simulink subsystem "EV3_Logic"  (R2020a)
settings: Solver=VariableStepAuto  StartTime=0.0  StopTime=10.0  RelTol=1e-3
values from neighbouring files (symbols this model uses):
  track = [1.6187 1.6087 1.5987 1.5887 1.5787 1.5687 1.5587 1.5487 1.5387 1.5287 1.5187 1.5087 ... (4048 elements, 1012x4)]    [config.mat]    (also in gen_track.m = [line_b; turn_bl; line_l; turn_lc; line_c; turn_ct; line_t; )
libraries: simulink_extras x5, simulink x4, dspnetwork x4, fuzblock x2
settings Model: Creator=Duncan  LastModifiedBy=abatra2

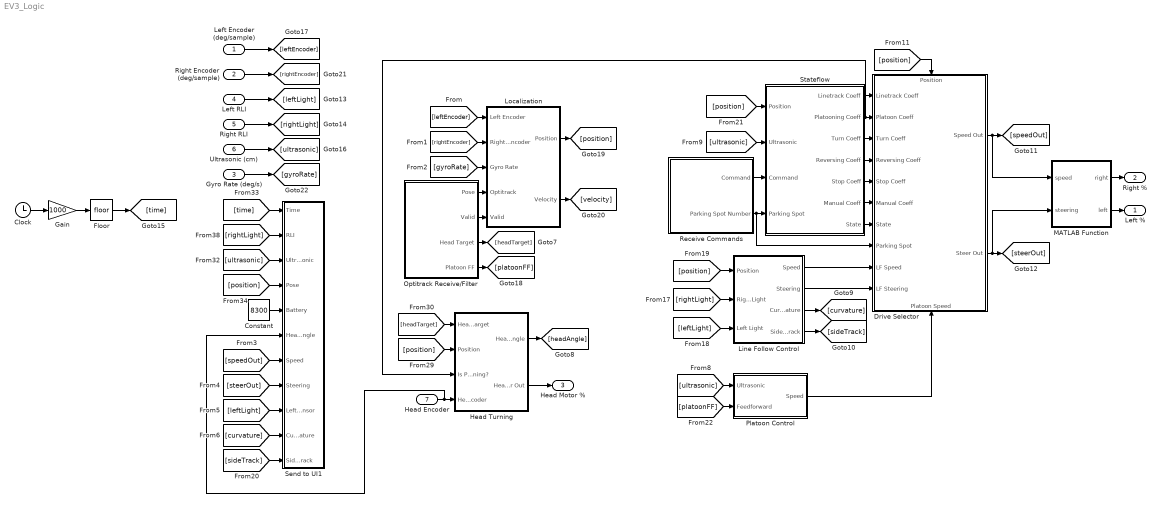
== system EV3_Logic ==
  Left Encoder (deg/sample) : Inport
  Right Encoder (deg/sample) : Inport  Port=2
  Gyro Rate (deg/s) : Inport  Port=3
  Left RLI : Inport  Port=4
  Right RLI : Inport  Port=5
  Ultrasonic (cm) : Inport  Port=6
  Head Encoder : Inport  Port=7
  Clock : Clock
  Constant : Constant  Value=8300
  Drive Selector : Subsystem
      settings: PortSchema="{\"entries\":[{\"content\":{\"sides\":[{\"content\":{\"connectorIds\":[\"In1\",\"In2\",\"In3\",\"In4\",\"In5\",\"In6\",\"In7\",\"In8\",\"In9\",\"In10\"]},\"type\":\"ConnectorPlacement.EquallySpacedRectSide\",\"uuid\":\"ae307232-287c-4602-bc59-e7aee20cf720\"},{\"content\":{\"connectorIds\":[\"Out1\",\"Out2\"],\"side\":\"RIGHT\"},\"type\":\"ConnectorPlacement.EquallySpacedRectSide\",\"uuid\":\"2cae2544-d808-4029-9530-a1f56251b9cd\"},{\"content\":{\"connectorIds\":[\"In11\"],\"side\":\"TOP\"},\"type\":\"ConnectorPlacement.EquallySpacedRectSide\",\"uuid\":\"bbc0be7b-0147-487e-824e-99eef1e06dcc\"},{\"content\":{\"connectorIds\":[\"In12\"],\"side\":\"BOTTOM\"},\"type\":\"ConnectorPlacement.EquallySpacedRectSide\",\"uuid\":\"b1fbed80-afe2-48db-af11-c85938407aae\"}]},\"type\":\"ConnectorPlacement.EquallySpacedConnector\",\"uuid\":\"38f7d747-6147-4f1b-8575-02c2e0fe0660\"}],\"packageUris\":[\"http://schema.mathworks.com/mf0/Connector/19700101\"],\"version\":\"1.0\"}"
  Floor : Rounding
  Gain : Gain  Gain=1000
  Head Turning : Subsystem
  Line Follow Control : Subsystem
  Localization : Subsystem
  MATLAB Function : MATLAB Function  TreatAsAtomicUnit=on
  Optitrack Receive/Filter : Subsystem
  Platoon Control : Subsystem
  Receive Commands : Subsystem
  Send to UI1 : Subsystem
  Stateflow : Subsystem
  Left % : Outport
  Right % : Outport  Port=2
  Head Motor % : Outport  Port=3
  wires:
  Ultrasonic (cm)/1 -> [ultrasonic]
  Right RLI/1 -> [rightLight]
  Left Encoder (deg/sample)/1 -> [leftEncoder]
  Right Encoder (deg/sample)/1 -> [rightEncoder]
  Left RLI/1 -> [leftLight]
  Gyro Rate (deg/s)/1 -> [gyroRate]
  Drive Selector/1(Speed Out) -> MATLAB Function/1(speed), [speedOut]
  Drive Selector/2(Steer Out) -> MATLAB Function/2(steering), [steerOut]
  Platoon Control/1(Speed) -> Drive Selector/12(Platoon Speed)
  Line Follow Control/4(Side Track) -> [sideTrack]
  Line Follow Control/3(Curvature) -> [curvature]
  Line Follow Control/2(Steering) -> Drive Selector/10(LF Steering)
  Line Follow Control/1(Speed) -> Drive Selector/9(LF Speed)
  Stateflow/2(Platooning Coeff) -> Drive Selector/2(Platoon Coeff), Head Turning/3(Is Platooning?)
  [ultrasonic] -> Platoon Control/1(Ultrasonic)
  [platoonFF] -> Platoon Control/2(Feedforward)
  Receive Commands/2(Parking Spot Number) -> Stateflow/4(Parking Spot), Drive Selector/8(Parking Spot)
  [ultrasonic] -> Stateflow/2(Ultrasonic)
  [position] -> Stateflow/1(Position)
  [sideTrack] -> Send to UI1/11(Side Track)
  [curvature] -> Send to UI1/10(Curvature)
  [leftLight] -> Send to UI1/9(Left Sensor)
  [steerOut] -> Send to UI1/8(Steering)
  [speedOut] -> Send to UI1/7(Speed)
  [position] -> Send to UI1/4(Pose)
  Stateflow/3(Turn Coeff) -> Drive Selector/3(Turn Coeff)
  [position] -> Drive Selector/11(Position)
  Localization/1(Position) -> [position]
  [leftEncoder] -> Localization/1(Left Encoder)
  Head Turning/1(Head Angle) -> [headAngle]
  Optitrack Receive/Filter/1(Pose) -> Localization/4(Optitrack)
  Stateflow/7(State) -> Drive Selector/7(State)
  Stateflow/5(Stop Coeff) -> Drive Selector/5(Stop Coeff)
  [rightEncoder] -> Localization/2(Right Encoder)
  [leftLight] -> Line Follow Control/3(Left Light)
  Stateflow/4(Reversing Coeff) -> Drive Selector/4(Reversing Coeff)
  [position] -> Head Turning/2(Position)
  [rightLight] -> Send to UI1/2(RLI)
  Localization/2(Velocity) -> [velocity]
  [time] -> Send to UI1/1(Time)
  [headTarget] -> Head Turning/1(Head Target)
  [ultrasonic] -> Send to UI1/3(Ultrasonic)
  Stateflow/1(Linetrack Coeff) -> Drive Selector/1(Linetrack Coeff)
  Optitrack Receive/Filter/2(Valid) -> Localization/5(Valid)
  [rightLight] -> Line Follow Control/2(Right Light)
  [gyroRate] -> Localization/3(Gyro Rate)
  Receive Commands/1(Command) -> Stateflow/3(Command)
  Head Turning/2(Head Motor Out) -> Head Motor %/1
  Head Encoder/1 -> Head Turning/4(Head Encoder), Send to UI1/6(Head Angle)
  Clock/1 -> Gain/1
  Gain/1 -> Floor/1
  Floor/1 -> [time]
  Optitrack Receive/Filter/3(Head Target) -> [headTarget]
  [position] -> Line Follow Control/1(Position)
  Optitrack Receive/Filter/4(Platoon FF) -> [platoonFF]
  Stateflow/6(Manual Coeff) -> Drive Selector/6(Manual Coeff)
  MATLAB Function/1(right) -> Right %/1
  MATLAB Function/2(left) -> Left %/1
  Constant/1 -> Send to UI1/5(Battery)

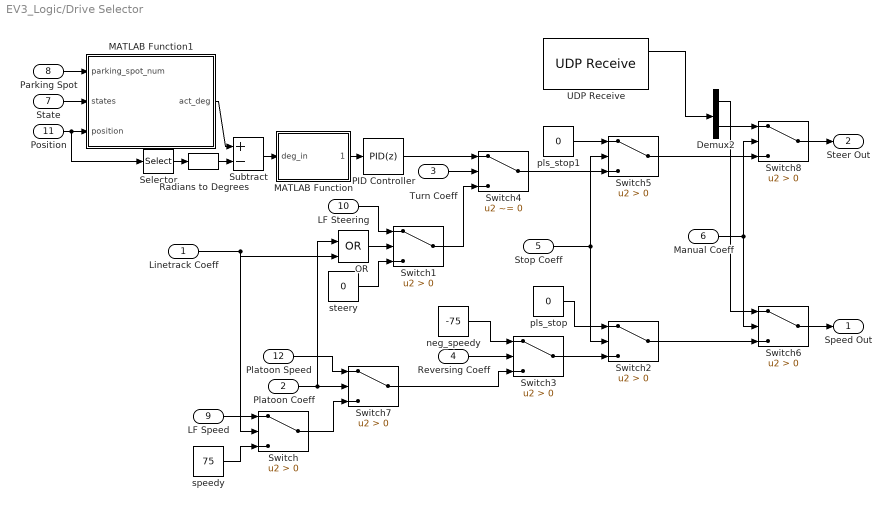
== system EV3_Logic/Drive Selector ==
  Linetrack Coeff : Inport
  Platoon Coeff : Inport  Port=2
  Turn Coeff : Inport  Port=3
  Reversing Coeff : Inport  Port=4
  Stop Coeff : Inport  Port=5
  Manual Coeff : Inport  Port=6
  State : Inport  Port=7
  Parking Spot : Inport  Port=8
  LF Speed : Inport  Port=9
  LF Steering : Inport  Port=10
  Position : Inport  Port=11
  Platoon Speed : Inport  Port=12
  Demux2 : Demux  Outputs=2
  MATLAB Function : MATLAB Function  TreatAsAtomicUnit=on
  MATLAB Function1 : MATLAB Function  TreatAsAtomicUnit=on
  OR : Logic  Operator=OR  IconShape=distinctive  AllPortsSameDT=off  OutDataTypeStr=boolean
  PID Controller : simulink/Continuous/PID Controller  Controller=PID  Form=Parallel  TimeDomain=Discrete-time  UseExternalTs=off  SampleTime=-1  IntegratorMethod=Forward Euler  FilterMethod=Forward Euler  ControllerParametersSource=internal  P=1  I=0  D=0  UseFilter=off  N=100  TunerSelectOption=Transfer Function Based (PID Tuner App)  InitialConditionSource=internal  InitialConditionForIntegrator=0  InitialConditionForFilter=0  DifferentiatorICPrevScaledInput=0  ExternalReset=none  TrackingMode=off  Kt=1  LimitOutput=off  UpperSaturationLimit=inf  LowerSaturationLimit=-inf  LinearizeAsGain=on  AntiWindupMode=none  Kb=1  POutMin=[]  POutMax=[]  IOutMin=[]  IOutMax=[]  DOutMin=[]  DOutMax=[]  NOutMin=[]  NOutMax=[]  SumOutMin=[]  SumOutMax=[]  SaturationOutMin=[]  SaturationOutMax=[]  PParamMin=[]  PParamMax=[]  IParamMin=[]  IParamMax=[]  DParamMin=[]  DParamMax=[]  NParamMin=[]  NParamMax=[]  KbParamMin=[]  KbParamMax=[]  KtParamMin=[]  KtParamMax=[]  KbOutMin=[]  KbOutMax=[]  KtOutMin=[]  KtOutMax=[]  IntegratorOutMin=[]  IntegratorOutMax=[]  FilterOutMin=[]  FilterOutMax=[]  SumI1OutMin=[]  SumI1OutMax=[]  SumI2OutMin=[]  SumI2OutMax=[]  SumI3OutMin=[]  SumI3OutMax=[]  SumI4OutMin=[]  SumI4OutMax=[]  SumDOutMin=[]  SumDOutMax=[]  DifferentiatorOutMin=[]  DifferentiatorOutMax=[]  FilterDiffOutCoefMin=[]  FilterDiffOutCoefMax=[]  ReciprocalOutMin=[]  ReciprocalOutMax=[]  SumDenOutMin=[]  SumDenOutMax=[]  SumNumOutMin=[]  SumNumOutMax=[]  DivideOutMin=[]  DivideOutMax=[]  UdiffTsProdOutMin=[]  UdiffTsProdOutMax=[]  NTsProdOutMin=[]  NTsProdOutMax=[]  UintegralTsProdOutMin=[]  UintegralTsProdOutMax=[]  UngainTsProdOutMin=[]  UngainTsProdOutMax=[]  IntegratorContinuousStateAttributes=''  IntegratorStateMustResolveToSignalObject=off  IntegratorRTWStateStorageClass=Auto  FilterContinuousStateAttributes=''  FilterStateMustResolveToSignalObject=off  FilterRTWStateStorageClass=Auto  ParallelPVariant=InternalParameters  IdealPVariant=Disabled  IVariant=InternalParameters  DVariant=InternalParameters  IntegratorVariant=Discrete  SatVariant=Disabled  AWVariant=Passthrough  PCopyVariant=Disabled  TRVariant=Disabled  FdbkBlocksVariant=Forward  IdealPFdbkVariant=Disabled  SatFdbkVariant=Disabled  DerivativeFilterVariant=Differentiator  NVariant=Passthrough  NCopyVariant=Disabled_SignalSpec  FilterICVariant=InternalICsDifferentiator  IntegratorICVariant=InternalICs  ExternalResetVariant=Disabled  TRSumVariant=Passthrough  SumFdbkVariant=Disabled  SumVariant=Sum_PID  TsampFilterVariant=InternalTs  TsampNgainVariant=Passthrough  TsampIntegralVariant=Passthrough
  Radians to Degrees : simulink_extras/Transformations/Radians to Degrees
  Selector : Selector  InputPortWidth=3  IndexOptions=Index vector (dialog)  Indices=[3]  OutputSizes=1
  Subtract : Sum  Inputs=+-
  Switch{,1..3,5..8} (8 alike) : Switch  Criteria=u2 > Threshold
  Switch4 : Switch  Criteria=u2 ~= 0
  UDP Receive : dspnetwork/UDP Receive  localURL='0.0.0.0'  localPort=joystickRXPort  remoteURL='0.0.0.0'  remotePort=-1  recvBufferSize=384  dims=2  signalDatatype=single  isComplex=off  isVarSize=off  showBlockingTime=off  blockingTime=0  sampletime=0.01  blockPlatform=[]
  neg_speedy : Constant  Value=-75
  pls_stop : Constant  Value=0
  pls_stop1 : Constant  Value=0
  speedy : Constant  Value=75
  steery : Constant  Value=0
  Speed Out : Outport
  Steer Out : Outport  Port=2
  wires:
  Platoon Speed/1 -> Switch7/1
  pls_stop1/1 -> Switch5/1
  Selector/1 -> Radians to Degrees/1
  Switch/1 -> Switch7/3
  Switch7/1 -> Switch3/3
  Linetrack Coeff/1 -> OR/2, Switch/2
  Platoon Coeff/1 -> Switch7/2, OR/1
  OR/1 -> Switch1/2
  MATLAB Function1/1(act_deg) -> Subtract/1
  neg_speedy/1 -> Switch3/1
  Switch4/1 -> Switch5/3
  Position/1 -> MATLAB Function1/3(position), Selector/1
  State/1 -> MATLAB Function1/2(states)
  Reversing Coeff/1 -> Switch3/2
  Parking Spot/1 -> MATLAB Function1/1(parking_spot_num)
  Radians to Degrees/1 -> Subtract/2
  MATLAB Function/1(deg_out) -> PID Controller/1
  Subtract/1 -> MATLAB Function/1(deg_in)
  PID Controller/1 -> Switch4/1
  Turn Coeff/1 -> Switch4/2
  pls_stop/1 -> Switch2/1
  Stop Coeff/1 -> Switch5/2, Switch2/2
  Switch3/1 -> Switch2/3
  Switch1/1 -> Switch4/3
  speedy/1 -> Switch/3
  steery/1 -> Switch1/3
  LF Steering/1 -> Switch1/1
  LF Speed/1 -> Switch/1
  UDP Receive/1 -> Demux2/1
  Switch5/1 -> Switch8/3
  Switch2/1 -> Switch6/3
  Manual Coeff/1 -> Switch8/2, Switch6/2
  Switch8/1 -> Steer Out/1
  Switch6/1 -> Speed Out/1
  Demux2/2 -> Switch8/1
  Demux2/1 -> Switch6/1

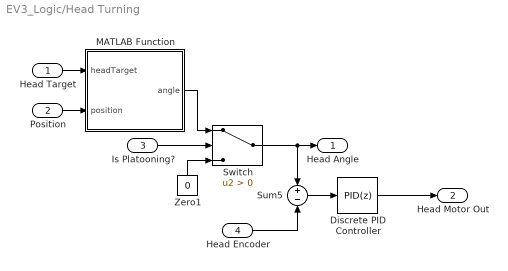
== system EV3_Logic/Head Turning ==
  Head Target : Inport
  Position : Inport  Port=2
  Is Platooning? : Inport  Port=3
  Head Encoder : Inport  Port=4
  Discrete PID Controller : simulink/Continuous/PID Controller  Controller=PID  Form=Parallel  TimeDomain=Discrete-time  UseExternalTs=off  SampleTime=-1  IntegratorMethod=Forward Euler  FilterMethod=Forward Euler  ControllerParametersSource=internal  P=1  I=1  D=0  UseFilter=off  N=100  TunerSelectOption=Transfer Function Based (PID Tuner App)  InitialConditionSource=internal  InitialConditionForIntegrator=0  InitialConditionForFilter=0  DifferentiatorICPrevScaledInput=0  ExternalReset=none  TrackingMode=off  Kt=1  LimitOutput=off  UpperSaturationLimit=inf  LowerSaturationLimit=-inf  LinearizeAsGain=off  AntiWindupMode=none  Kb=1  POutMin=[]  POutMax=[]  IOutMin=[]  IOutMax=[]  DOutMin=[]  DOutMax=[]  NOutMin=[]  NOutMax=[]  SumOutMin=[]  SumOutMax=[]  SaturationOutMin=[]  SaturationOutMax=[]  PParamMin=[]  PParamMax=[]  IParamMin=[]  IParamMax=[]  DParamMin=[]  DParamMax=[]  NParamMin=[]  NParamMax=[]  KbParamMin=[]  KbParamMax=[]  KtParamMin=[]  KtParamMax=[]  KbOutMin=[]  KbOutMax=[]  KtOutMin=[]  KtOutMax=[]  IntegratorOutMin=[]  IntegratorOutMax=[]  FilterOutMin=[]  FilterOutMax=[]  SumI1OutMin=[]  SumI1OutMax=[]  SumI2OutMin=[]  SumI2OutMax=[]  SumI3OutMin=[]  SumI3OutMax=[]  SumI4OutMin=[]  SumI4OutMax=[]  SumDOutMin=[]  SumDOutMax=[]  DifferentiatorOutMin=[]  DifferentiatorOutMax=[]  FilterDiffOutCoefMin=[]  FilterDiffOutCoefMax=[]  ReciprocalOutMin=[]  ReciprocalOutMax=[]  SumDenOutMin=[]  SumDenOutMax=[]  SumNumOutMin=[]  SumNumOutMax=[]  DivideOutMin=[]  DivideOutMax=[]  UdiffTsProdOutMin=[]  UdiffTsProdOutMax=[]  NTsProdOutMin=[]  NTsProdOutMax=[]  UintegralTsProdOutMin=[]  UintegralTsProdOutMax=[]  UngainTsProdOutMin=[]  UngainTsProdOutMax=[]  IntegratorContinuousStateAttributes=''  IntegratorStateMustResolveToSignalObject=off  IntegratorRTWStateStorageClass=Auto  FilterContinuousStateAttributes=''  FilterStateMustResolveToSignalObject=off  FilterRTWStateStorageClass=Auto  ParallelPVariant=InternalParameters  IdealPVariant=Disabled  IVariant=InternalParameters  DVariant=InternalParameters  IntegratorVariant=Discrete  SatVariant=Disabled  AWVariant=Passthrough  PCopyVariant=Disabled  TRVariant=Disabled  FdbkBlocksVariant=Forward  IdealPFdbkVariant=Disabled  SatFdbkVariant=Disabled  DerivativeFilterVariant=Differentiator  NVariant=Passthrough  NCopyVariant=Disabled_SignalSpec  FilterICVariant=InternalICsDifferentiator  IntegratorICVariant=InternalICs  ExternalResetVariant=Disabled  TRSumVariant=Passthrough  SumFdbkVariant=Disabled  SumVariant=Sum_PID  TsampFilterVariant=InternalTs  TsampNgainVariant=Passthrough  TsampIntegralVariant=Passthrough
  MATLAB Function : MATLAB Function  TreatAsAtomicUnit=on
  Sum5 : Sum  Inputs=+|-
  Switch : Switch  Criteria=u2 > Threshold
  Zero1 : Constant  Value=0  OutDataTypeStr=Inherit: Inherit via back propagation
  Head Angle : Outport
  Head Motor Out : Outport  Port=2
  wires:
  Is Platooning?/1 -> Switch/2
  MATLAB Function/1(angle) -> Switch/1
  Head Target/1 -> MATLAB Function/1(headTarget)
  Discrete PID Controller/1 -> Head Motor Out/1
  Switch/1 -> Sum5/1, Head Angle/1
  Zero1/1 -> Switch/3
  Sum5/1 -> Discrete PID Controller/1
  Position/1 -> MATLAB Function/2(position)
  Head Encoder/1 -> Sum5/2

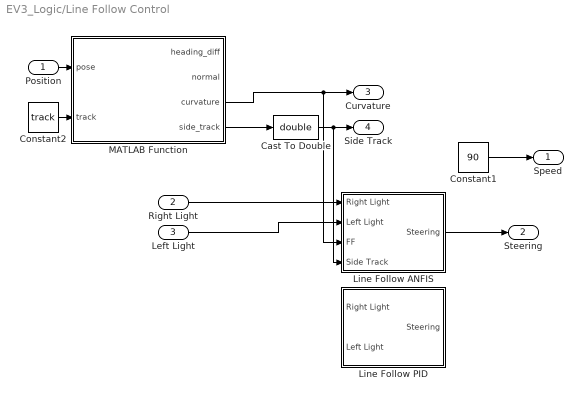
== system EV3_Logic/Line Follow Control ==
  Position : Inport
  Right Light : Inport  Port=2
  Left Light : Inport  Port=3
  Cast To Double : DataTypeConversion  OutDataTypeStr=double
  Constant1 : Constant  Value=90
  Constant2 : Constant  Value=track
  Line Follow ANFIS : Subsystem
  Line Follow PID : Subsystem
  MATLAB Function : MATLAB Function  TreatAsAtomicUnit=on
  Speed : Outport
  Steering : Outport  Port=2
  Curvature : Outport  Port=3
  Side Track : Outport  Port=4
  wires:
  Constant1/1 -> Speed/1
  Cast To Double/1 -> Line Follow ANFIS/4(Side Track), Side Track/1
  MATLAB Function/3(curvature) -> Line Follow ANFIS/3(FF), Curvature/1
  Position/1 -> MATLAB Function/1(pose)
  MATLAB Function/4(side_track) -> Cast To Double/1
  Constant2/1 -> MATLAB Function/2(track)
  Right Light/1 -> Line Follow ANFIS/1(Right Light)
  Left Light/1 -> Line Follow ANFIS/2(Left Light)
  Line Follow ANFIS/1(Steering) -> Steering/1

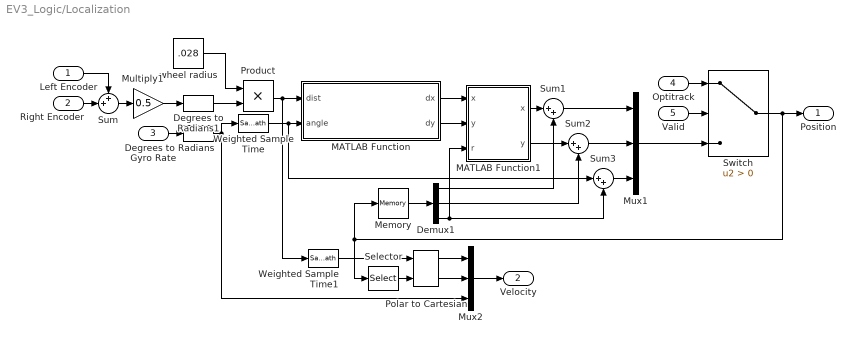
== system EV3_Logic/Localization ==
  Left Encoder : Inport
  Right Encoder : Inport  Port=2
  Gyro Rate : Inport  Port=3
  Optitrack : Inport  Port=4
  Valid : Inport  Port=5
  Degrees to Radians : simulink_extras/Transformations/Degrees to Radians
  Degrees to Radians1 : simulink_extras/Transformations/Degrees to Radians
  Demux1 : Demux  Outputs=3
  MATLAB Function : MATLAB Function  TreatAsAtomicUnit=on
  MATLAB Function1 : MATLAB Function  TreatAsAtomicUnit=on
  Memory : Memory
  Multiply1 : Gain  Gain=0.5
  Mux1 : Mux  Inputs=3
  Mux2 : Mux  Inputs=3
  Polar to Cartesian : simulink_extras/Transformations/Polar to Cartesian
      settings: SourceProductBaseCode=SL
  Product : Product
  Selector : Selector  InputPortWidth=3  IndexOptions=Index vector (dialog)  Indices=[3]  OutputSizes=1
  Sum : Sum  Inputs=++|
  Sum1 : Sum  Inputs=|++
  Sum2 : Sum  Inputs=|++
  Sum3 : Sum  Inputs=|++
  Switch : Switch  Criteria=u2 > Threshold
  Weighted Sample Time : SampleTimeMath  TsampMathOp=*
  Weighted Sample Time1 : SampleTimeMath  TsampMathOp=/
  wheel radius : Constant  Value=.028
  Position : Outport
  Velocity : Outport  Port=2
  wires:
  wheel radius/1 -> Product/1
  Degrees to Radians1/1 -> Product/2
  Product/1 -> MATLAB Function/1(dist), Weighted Sample Time1/1
  Multiply1/1 -> Degrees to Radians1/1
  Weighted Sample Time1/1 -> Polar to Cartesian/1
  Mux2/1 -> Velocity/1
  Polar to Cartesian/2 -> Mux2/2
  Polar to Cartesian/1 -> Mux2/1
  Selector/1 -> Polar to Cartesian/2
  Switch/1 -> Selector/1, Memory/1, Position/1
  Optitrack/1 -> Switch/1
  Valid/1 -> Switch/2
  Mux1/1 -> Switch/3
  Weighted Sample Time/1 -> MATLAB Function/2(angle), Sum3/1
  Degrees to Radians/1 -> Weighted Sample Time/1, Mux2/3
  Gyro Rate/1 -> Degrees to Radians/1
  Right Encoder/1 -> Sum/2
  Left Encoder/1 -> Sum/1
  Sum3/1 -> Mux1/3
  Sum2/1 -> Mux1/2
  Sum1/1 -> Mux1/1
  Demux1/2 -> Sum2/2
  Demux1/1 -> Sum1/2
  MATLAB Function1/2(y) -> Sum2/1
  MATLAB Function1/1(x) -> Sum1/1
  Demux1/3 -> Sum3/2, MATLAB Function1/3(r)
  Memory/1 -> Demux1/1
  MATLAB Function/2(dy) -> MATLAB Function1/2("y ")
  MATLAB Function/1(dx) -> MATLAB Function1/1("x ")
  Sum/1 -> Multiply1/1

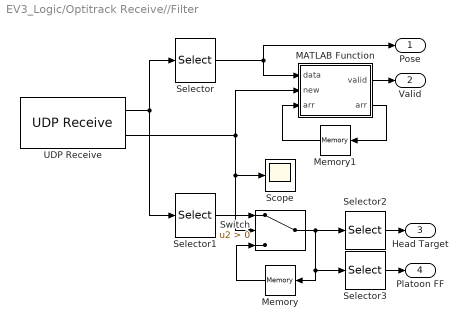
== system EV3_Logic/Optitrack Receive//Filter ==
  MATLAB Function : MATLAB Function  TreatAsAtomicUnit=on
  Memory : Memory
  Memory1 : Memory
  Scope : Scope
  Selector : Selector  InputPortWidth=6  IndexOptions=Index vector (dialog)  Indices=[1:3]  OutputSizes=1
  Selector1 : Selector  InputPortWidth=6  IndexOptions=Index vector (dialog)  Indices=[4:6]  OutputSizes=1
  Selector2 : Selector  InputPortWidth=3  IndexOptions=Index vector (dialog)  Indices=[1:2]  OutputSizes=1
  Selector3 : Selector  InputPortWidth=3  IndexOptions=Index vector (dialog)  Indices=[3]  OutputSizes=1
  Switch : Switch  Criteria=u2 > Threshold
  UDP Receive : dspnetwork/UDP Receive  localURL='0.0.0.0'  localPort=dataRXPort  remoteURL='0.0.0.0'  remotePort=-1  recvBufferSize=384  dims=6  signalDatatype=single  isComplex=off  isVarSize=off  showBlockingTime=off  blockingTime=0  sampletime=0.01  blockPlatform=[]
  Pose : Outport
  Valid : Outport  Port=2
  Head Target : Outport  Port=3
  Platoon FF : Outport  Port=4
  wires:
  UDP Receive/2 -> MATLAB Function/2(new), Switch/2, Scope/1
  Selector3/1 -> Platoon FF/1
  Selector2/1 -> Head Target/1
  UDP Receive/1 -> Selector1/1, Selector/1
  Selector1/1 -> Switch/1
  Switch/1 -> Memory/1, Selector3/1, Selector2/1
  Memory/1 -> Switch/3
  Selector/1 -> MATLAB Function/1(data), Pose/1
  Memory1/1 -> MATLAB Function/3("arr ")
  MATLAB Function/2(arr) -> Memory1/1
  MATLAB Function/1(valid) -> Valid/1

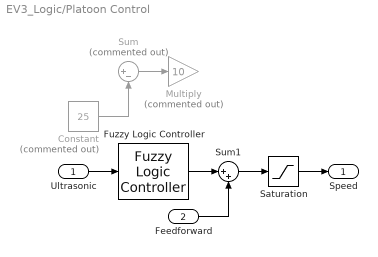
== system EV3_Logic/Platoon Control ==
  Ultrasonic : Inport
  Feedforward : Inport  Port=2
  Constant : Constant  Commented=on  Value=25
  Fuzzy Logic Controller : fuzblock/Fuzzy Logic  Controller  FIS='platoon-anfis.fis'  OutputSampleNumber=101  DataType=double  FuzzifiedInputs=off  RuleFiringStrengths=off  RuleOutputs=off  AggregatedOutputs=off  SimulateUsing=Code generation  OutOfRangeInputValueMessage=none  NoRuleFiredMessage=none  EmptyOutputFuzzySetMessage=none
  Multiply : Gain  Commented=on  Gain=10
  Saturation : Saturate  UpperLimit=100  LowerLimit=-100
  Sum : Sum  Commented=on  Inputs=|+-
  Sum1 : Sum  Inputs=|++
  Speed : Outport
  wires:
  Fuzzy Logic Controller/1 -> Sum1/1
  Ultrasonic/1 -> Fuzzy Logic Controller/1
  Feedforward/1 -> Sum1/2
  Sum1/1 -> Saturation/1
  Constant/1 -> Sum/2
  Saturation/1 -> Speed/1
  Sum/1 -> Multiply/1

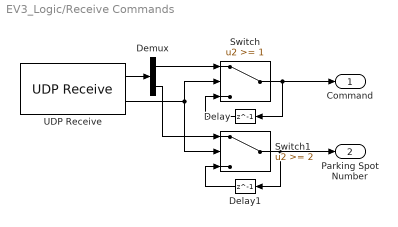
== system EV3_Logic/Receive Commands ==
  Delay : Delay  DelayLength=1  InitialCondition=0
  Delay1 : Delay  DelayLength=1  InitialCondition=0
  Demux : Demux  Outputs=2
  Switch : Switch  Threshold=1
  Switch1 : Switch  Threshold=2
  UDP Receive : dspnetwork/UDP Receive  localURL='0.0.0.0'  localPort=cmdPort  remoteURL='0.0.0.0'  remotePort=-1  recvBufferSize=384  dims=2  signalDatatype=uint8  isComplex=off  isVarSize=off  showBlockingTime=off  blockingTime=0  sampletime=0.01  blockPlatform=[]
  Command : Outport
  Parking Spot Number : Outport  Port=2
  wires:
  Demux/2 -> Switch1/1
  Delay1/1 -> Switch1/3
  Switch1/1 -> Delay1/1, Parking Spot Number/1
  Delay/1 -> Switch/3
  Switch/1 -> Delay/1, Command/1
  Demux/1 -> Switch/1
  UDP Receive/1 -> Demux/1
  UDP Receive/2 -> Switch1/2, Switch/2

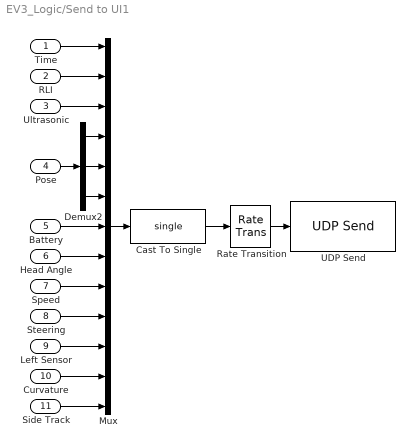
== system EV3_Logic/Send to UI1 ==
  Time : Inport
  RLI : Inport  Port=2
  Ultrasonic : Inport  Port=3
  Pose : Inport  Port=4
  Battery : Inport  Port=5
  Head Angle : Inport  Port=6
  Speed : Inport  Port=7
  Steering : Inport  Port=8
  Left Sensor : Inport  Port=9
  Curvature : Inport  Port=10
  Side Track : Inport  Port=11
  Cast To Single : DataTypeConversion  OutDataTypeStr=single
  Demux2 : Demux  Outputs=3
  Mux : Mux  Inputs=13
  Rate Transition : RateTransition  OutPortSampleTime=.04
  UDP Send : dspnetwork/UDP Send  remoteURL='127.0.0.1'  remotePort=dataTXPort  localURL='0.0.0.0'  localPortSource=Automatically determine  localPort=-1  sendBufferSize=8192  sampletime=-1  blockPlatform=[]  separateLengthPort=0
  wires:
  Side Track/1 -> Mux/13
  Curvature/1 -> Mux/12
  Left Sensor/1 -> Mux/11
  Steering/1 -> Mux/10
  Head Angle/1 -> Mux/8
  Speed/1 -> Mux/9
  Time/1 -> Mux/1
  Cast To Single/1 -> Rate Transition/1
  RLI/1 -> Mux/2
  Demux2/3 -> Mux/6
  Demux2/2 -> Mux/5
  Mux/1 -> Cast To Single/1
  Battery/1 -> Mux/7
  Pose/1 -> Demux2/1
  Ultrasonic/1 -> Mux/3
  Demux2/1 -> Mux/4
  Rate Transition/1 -> UDP Send/1

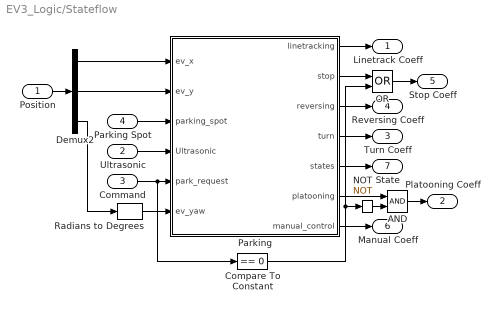
== system EV3_Logic/Stateflow ==
  Position : Inport
  Ultrasonic : Inport  Port=2
  Command : Inport  Port=3
  Parking Spot : Inport  Port=4
  AND : Logic  IconShape=distinctive  AllPortsSameDT=off  OutDataTypeStr=boolean
  Compare To Constant : simulink/Logic and Bit Operations/Compare To Constant  relop===  const=0  OutDataTypeStr=boolean
  Demux2 : Demux  Outputs=3
  NOT : Logic  Operator=NOT  IconShape=distinctive  AllPortsSameDT=off  OutDataTypeStr=boolean
  OR : Logic  Operator=OR  IconShape=distinctive  AllPortsSameDT=off  OutDataTypeStr=boolean
  Parking : Stateflow chart  TreatAsAtomicUnit=on
  Radians to Degrees : simulink_extras/Transformations/Radians to Degrees
  Linetrack Coeff : Outport
  Platooning Coeff : Outport  Port=2
  Turn Coeff : Outport  Port=3
  Reversing Coeff : Outport  Port=4
  Stop Coeff : Outport  Port=5
  Manual Coeff : Outport  Port=6
  State : Outport  Port=7
  wires:
  Command/1 -> Compare To Constant/1, Parking/5(park_request)
  Radians to Degrees/1 -> Parking/6(ev_yaw)
  Parking/5(states) -> State/1
  Position/1 -> Demux2/1
  Parking/4(turn) -> Turn Coeff/1
  Demux2/1 -> Parking/1(ev_x)
  Parking Spot/1 -> Parking/3(parking_spot)
  Parking/3(reversing) -> Reversing Coeff/1
  Demux2/2 -> Parking/2(ev_y)
  Parking/1(linetracking) -> Linetrack Coeff/1
  Ultrasonic/1 -> Parking/4(Ultrasonic)
  Demux2/3 -> Radians to Degrees/1
  Parking/7(manual_control) -> Manual Coeff/1
  OR/1 -> Stop Coeff/1
  Parking/2(stop) -> OR/1
  Compare To Constant/1 -> NOT/1, OR/2
  Parking/6(platooning) -> AND/1
  AND/1 -> Platooning Coeff/1
  NOT/1 -> AND/2

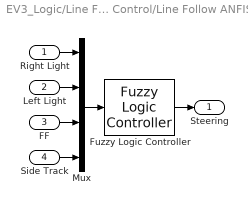
== system EV3_Logic/Line Follow Control/Line Follow ANFIS ==
  Right Light : Inport
  Left Light : Inport  Port=2
  FF : Inport  Port=3
  Side Track : Inport  Port=4
  Fuzzy Logic Controller : fuzblock/Fuzzy Logic  Controller  FIS='linefollow-anfis.fis'  OutputSampleNumber=101  DataType=double  FuzzifiedInputs=off  RuleFiringStrengths=off  RuleOutputs=off  AggregatedOutputs=off  SimulateUsing=Code generation  OutOfRangeInputValueMessage=warning  NoRuleFiredMessage=warning  EmptyOutputFuzzySetMessage=warning
  Mux : Mux
  Steering : Outport
  wires:
  Right Light/1 -> Mux/1
  Left Light/1 -> Mux/2
  FF/1 -> Mux/3
  Side Track/1 -> Mux/4
  Mux/1 -> Fuzzy Logic Controller/1
  Fuzzy Logic Controller/1 -> Steering/1

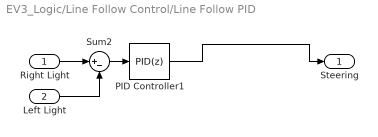
== system EV3_Logic/Line Follow Control/Line Follow PID ==
  Right Light : Inport
  Left Light : Inport  Port=2
  PID Controller1 : simulink/Continuous/PID Controller  Controller=PID  Form=Parallel  TimeDomain=Discrete-time  UseExternalTs=off  SampleTime=-1  IntegratorMethod=Forward Euler  FilterMethod=Forward Euler  ControllerParametersSource=internal  P=2  I=0.1  D=0.1  UseFilter=off  N=100  TunerSelectOption=Transfer Function Based (PID Tuner App)  InitialConditionSource=internal  InitialConditionForIntegrator=0  InitialConditionForFilter=0  DifferentiatorICPrevScaledInput=0  ExternalReset=none  TrackingMode=off  Kt=1  LimitOutput=off  UpperSaturationLimit=inf  LowerSaturationLimit=-inf  LinearizeAsGain=on  AntiWindupMode=none  Kb=1  POutMin=[]  POutMax=[]  IOutMin=[]  IOutMax=[]  DOutMin=[]  DOutMax=[]  NOutMin=[]  NOutMax=[]  SumOutMin=[]  SumOutMax=[]  SaturationOutMin=[]  SaturationOutMax=[]  PParamMin=[]  PParamMax=[]  IParamMin=[]  IParamMax=[]  DParamMin=[]  DParamMax=[]  NParamMin=[]  NParamMax=[]  KbParamMin=[]  KbParamMax=[]  KtParamMin=[]  KtParamMax=[]  KbOutMin=[]  KbOutMax=[]  KtOutMin=[]  KtOutMax=[]  IntegratorOutMin=[]  IntegratorOutMax=[]  FilterOutMin=[]  FilterOutMax=[]  SumI1OutMin=[]  SumI1OutMax=[]  SumI2OutMin=[]  SumI2OutMax=[]  SumI3OutMin=[]  SumI3OutMax=[]  SumI4OutMin=[]  SumI4OutMax=[]  SumDOutMin=[]  SumDOutMax=[]  DifferentiatorOutMin=[]  DifferentiatorOutMax=[]  FilterDiffOutCoefMin=[]  FilterDiffOutCoefMax=[]  ReciprocalOutMin=[]  ReciprocalOutMax=[]  SumDenOutMin=[]  SumDenOutMax=[]  SumNumOutMin=[]  SumNumOutMax=[]  DivideOutMin=[]  DivideOutMax=[]  UdiffTsProdOutMin=[]  UdiffTsProdOutMax=[]  NTsProdOutMin=[]  NTsProdOutMax=[]  UintegralTsProdOutMin=[]  UintegralTsProdOutMax=[]  UngainTsProdOutMin=[]  UngainTsProdOutMax=[]  IntegratorContinuousStateAttributes=''  IntegratorStateMustResolveToSignalObject=off  IntegratorRTWStateStorageClass=Auto  FilterContinuousStateAttributes=''  FilterStateMustResolveToSignalObject=off  FilterRTWStateStorageClass=Auto  ParallelPVariant=InternalParameters  IdealPVariant=Disabled  IVariant=InternalParameters  DVariant=InternalParameters  IntegratorVariant=Discrete  SatVariant=Disabled  AWVariant=Passthrough  PCopyVariant=Disabled  TRVariant=Disabled  FdbkBlocksVariant=Forward  IdealPFdbkVariant=Disabled  SatFdbkVariant=Disabled  DerivativeFilterVariant=Differentiator  NVariant=Passthrough  NCopyVariant=Disabled_SignalSpec  FilterICVariant=InternalICsDifferentiator  IntegratorICVariant=InternalICs  ExternalResetVariant=Disabled  TRSumVariant=Passthrough  SumFdbkVariant=Disabled  SumVariant=Sum_PID  TsampFilterVariant=InternalTs  TsampNgainVariant=Passthrough  TsampIntegralVariant=Passthrough
  Sum2 : Sum  Inputs=|+-
  Steering : Outport
  wires:
  Sum2/1 -> PID Controller1/1
  Left Light/1 -> Sum2/2
  Right Light/1 -> Sum2/1
  PID Controller1/1 -> Steering/1

== matlab function EV3_Logic/Drive Selector/MATLAB Function ==
  data: deg_in input; deg_out output
function deg_out = remainder(deg_in)

deg_out = mod(deg_in+180,360)-180;

== matlab function EV3_Logic/Drive Selector/MATLAB Function1 ==
  data: parking_spot_num input; act_deg output; states input; position input
function act_deg = atan_me(parking_spot_num, states, position)

if parking_spot_num ==1 && states == 10
    degg = atan2(1.8-position(2), 0-position(1)); 
    
elseif parking_spot_num ==2 && states ==10
    degg = atan2(1.525 - position(2), 0-position(1));
    
elseif parking_spot_num ==3 && states == 10
    degg = atan2(1.1 - position(2), 0-position(1));
    
elseif parking_spot_num == 1 && states == 20
    %go to parking spot 1
    degg= atan2(1.6-position(2), -0.45-position(1)); 
%     degg = -168;
    
elseif parking_spot_num ==2 && states == 20
     %go to parking spot 2
    degg =atan2(1.2-position(2), -0.75-position(1)); 
%     degg = -165;
    
elseif parking_spot_num ==3 && states == 20 
    %go to parkin spot 3
    degg = atan2(0.80-position(2), -0.85-position(1)); 
%     degg = -150;
elseif parking_spot_num ~=0 && states == 30
    %complete parking and move angle to 180 degrees
    degg = pi; 
    
elseif parking_spot_num ~=0 && states == 40 
    %go to stop sign
    degg = atan2(0.525-position(2),0.0935-position(1)); 
    
elseif parking_spot_num ~=0 && states == 50
    degg = atan2(0.33 - position(2), -0.3 - position(1));
    %degg = -90; 
    
else
    degg = 0;
end 
act_deg = rad2deg(degg);
%act_deg = degg;

== matlab function EV3_Logic/Head Turning/MATLAB Function ==
  data: headTarget input; angle output; position input
function angle = headAngle(headTarget, position)

diff = headTarget - position(1:2);
angle = -double(rad2deg(atan2(diff(2),diff(1))-position(3)));
angle = mod(angle+180, 360) - 180;

== matlab function EV3_Logic/Line Follow Control/MATLAB Function ==
  data: pose input; track input; heading_diff output; normal output; curvature output; side_track output
function [heading_diff, normal, curvature, side_track]= region_info(pose,track)

sensor = pose(1:2) + 0.06*[cos(pose(3));sin(pose(3))];
[~,index] = min((track(:,1)-sensor(1)).^2 + (track(:,2)-sensor(2)).^2);

point = track(index,1:2)';
direction = track(index,3);
curvature = track(index,4);

heading_diff = direction - pose(3);
heading_diff = heading_diff - 2*pi*round(heading_diff/(2*pi));

normal = dot(sensor-point, [sin(direction); -cos(direction)]);

x = sensor(1);
% side_track = (x>0.057 && x<0.247) || (x>0.619 && x<0.713) ...
%              || (x>0.875 && x<0.969) || (x>1.333 && x<1.523);
% side_track = (x>0.007 && x<0.297) || (x>0.569 && x<0.763) ...
%              || (x>0.825 && x<1.019) || (x>1.283 && x<1.573);
side_track = (x>0.569 && x<0.763) || (x>0.825 && x<1.019) || (x>1.283 && x<1.573);

== matlab function EV3_Logic/Localization/MATLAB Function ==
  data: dx output; dist input; angle input; dy output
function [dx,dy] = arc_approximation(dist,angle)
    if angle == 0
        dx = dist;
        dy = 0;
    else
        dx = sin(angle) * dist / angle;
        dy = (1-cos(angle)) * dist / angle;
    end

== matlab function EV3_Logic/Localization/MATLAB Function1 ==
  data: x input; x output; y input; r input; y output
function [x,y] = rotate2d(x,y,r)
    rot = [cos(r) -sin(r); sin(r) cos(r)] * [x;y];
    x = rot(1);
    y = rot(2);

== matlab function EV3_Logic/MATLAB Function ==
  data: right output; speed input; left output; steering input
function [right, left]= toMotorSpeeds(speed, steering)

left = speed - steering;
right = speed + steering;

m = max(left,right);
if m > 100
    left = left - m + 100;
    right = right - m + 100;
end

== matlab function EV3_Logic/Optitrack Receive//Filter/MATLAB Function ==
  data: data input; new input; arr input; valid output boolean; arr output
function [valid, arr]= filter(data,new,arr)

valid = false;
if new
    arr = circshift(arr,1);
    arr(1) = data(3);
    d = diff(arr);
    d = d - 2*pi*round(d/(2*pi));
    valid = all(abs(d) < deg2rad(5), 'all');
end

== stateflow chart EV3_Logic/Stateflow/Parking ==
  settings: executeAtInitialization=1
  state Leader_Goto_Intersection
    entry:
    linetracking =1;
    platooning =0;
    reversing = 0;
    turn = 0;
    stop =0;
    states = 10000;
  state Follower_Goto_Intersection
    entry:
    linetracking = 0;
    platooning =1;
    reversing = 0;
    turn =0;
    stop =0;
    states = 01000;
  state Enter_ParkingArea
    %Turn car 90 degrees
    entry:
    linetracking = 0;
    platooning =0;
    reversing = 0;
    turn = -1;
    stop =0;
    states = 00010;
  state Find_ParkingSpot
    entry:
    linetracking = 0;
    platooning  =0;
    reversing = 0;
    turn =2;
    stop = 0;
    states = 00020;
    %turn = 2 means find park (step 2 in turning)
    %Use the center of the target values to solve for the desired yaw that we want
    % Parking Spot 1 : x_cent = -0.45 ; y_cent =  1.6
    %Parking Spot 2: x_cent = -0.75; y_cent = 1.2
    %Parking Spot 3: x_cent = -0.85; y_cent = 0.80
  state Parking
    entry:
    linetracking = 0;
    platooning = 0;
    reversing = 0;
    turn=3;
    stop = 0;
    states = 00030;
    %turn =3 means 180 degrees
    %parking means to slow down the motor speed,
    %and to use ultrasonic sensor to detect for wall to stop
    %If ultrasonic sensor reaches a range of values-->parked
  state Parked
    entry:
    linetracking = 0;
    platooning = 0;
    reversing = 0;
    turn=0;
    stop = 1;
    states = 00001;
    %stop the car
  state Manual_Control
    entry:
    manual_control = 1;
    states = 100000;
    exit:
    manual_control = 0;
  state Reverse_Out_Spot
    entry:
    linetracking = 0;
    platooning = 0;
    reversing = 1;
    turn = 0;
    stop = 0;
    states = 00100;
    %once we find coordinate spot b we can
    %get rid of line tracking
  state Goto_Stop_Sign
    entry:
    linetracking = 0;
    platooning =0;
    reversing = 0;
    turn = 4;
    stop = 0;
    states = 00040;
    %turn = 4 means parking sign angle
  state Turn_Car_toInter
    %turn car -90 degrees
    entry:
    linetracking = 0;
    platooning =0;
    reversing = 0;
    turn = 5;
    stop = 0;
    states = 00050;
  state Finished
    entry:
    linetracking = 1;
    platooning =0;
    reversing = 0;
    turn =0;
    stop = 0;
    states = 10000;
    %can continue to linetrack the path.
  Manual_Control -> Leader_Goto_Intersection : [park_request ~= 4]
  Finished -> Leader_Goto_Intersection [order 1]
  (default) -> Leader_Goto_Intersection
  Leader_Goto_Intersection -> Follower_Goto_Intersection [order 1] : [park_request ==2]
  Leader_Goto_Intersection -> Manual_Control [order 3] : [park_request == 4]
  Follower_Goto_Intersection -> Manual_Control [order 3] : [park_request == 4]
  Follower_Goto_Intersection -> Leader_Goto_Intersection [order 1] : [park_request ==1]
  Leader_Goto_Intersection -> Enter_ParkingArea [order 2] : [park_request == 3 && ev_x <= 0.2 && ev_x >= -0.2...
      |  && ev_y <=3 && ev_y >= 2 ]
  Follower_Goto_Intersection -> Enter_ParkingArea [order 2] : [park_request == 3 && ev_x <= 0.2 && ev_x >= -0.2...
      |  && ev_y <=3 && ev_y >= 2 ]
  Enter_ParkingArea -> Manual_Control [order 2] : [park_request == 4]
  Enter_ParkingArea -> Find_ParkingSpot [order 1] : [(ev_yaw <=-85 && ev_yaw>= -95)&&...
      | ((parking_spot ==1 && ev_x <=0.30 && ev_x >=-0.30 && ev_y<=1.9 && ev_y >= 1.7) ||...
      |  (parking_spot == 2 && ev_x <= 0.30 && ev_x>= -0.30 && ev_y<=1.6 && ev_y >= 1.45) ||...
      |  (parking_spot ==3 && ev_x <=0.30&& ev_x >= -0.30 && ev_y <=1.2 && ev_y >= 1))]
  Find_ParkingSpot -> Manual_Control [order 2] : [park_request == 4]
  Find_ParkingSpot -> Parking [order 1] : [(parking_spot ==1 && ev_x <= -0.40 && ev_x >= -0.50 && ev_y<=1.7...
      |  && ev_y >= 1.5) || (parking_spot == 2 && ev_x<=-0.70 && ev_x>=-0.80....
      |  && ev_y<=1.3 && ev_y >= 1.1) || (parking_spot ==3 ...
      | && ev_x <=-0.80 && ev_x>= -0.90 && ev_y>=0.70 && ev_y <=0.90)]
  Parking -> Manual_Control [order 2] : [park_request == 4]
  Parking -> Parked [order 1] : [Ultrasonic <= 15]
  Parked -> Manual_Control [order 2] : [park_request == 4]
  Parked -> Reverse_Out_Spot [order 1] : [park_request == 1 || park_request ==2]
  Turn_Car_toInter -> Manual_Control [order 2] : [park_request == 4]
  Goto_Stop_Sign -> Manual_Control [order 2] : [park_request == 4]
  Finished -> Manual_Control [order 2] : [park_request == 4]
  Reverse_Out_Spot -> Manual_Control [order 2] : [park_request == 4]
  Reverse_Out_Spot -> Goto_Stop_Sign [order 1] : [(parking_spot ==1 && ev_x <=0.30 && ev_x >=-0.30 ...
      | && ev_y<=1.9 && ev_y >= 1.4) || (parking_spot == 2 ...
      |   && ev_x <= 0.30 && ev_x>= -0.30 && ev_y<=1.3 ...
      | && ev_y >= 1) || (parking_spot ==3 && ev_x <=0.30...
      | && ev_x >= -0.30 && ev_y <=1 && ev_y >= 0.65)]
  Goto_Stop_Sign -> Turn_Car_toInter [order 1] : [ev_x <= 0.17 && ev_x >= 0.017...
      |  && ev_y >= 0.45 && ev_y <= 0.6]
  Turn_Car_toInter -> Finished [order 1] : [ev_x>=-0.5 && ev_x <= -0.10 && ev_y<=0.36 && ev_y >= 0.3 ]
  data: ev_x input; ev_y input; parking_spot input; Ultrasonic input; linetracking output double; stop output double; reversing output double; turn output double; states output double; park_request input; ev_yaw input; platooning output double; manual_control output double
